simulink library "everscale_lib"  (R2018b)
settings: Solver=VariableStepAuto  StartTime=0.0  StopTime=10.0  RelTol=1e-3
undefined symbols (not defined in the file or in its folder): lindi
libraries: filters_lib x1
settings Model: Creator=Ybeyer  LastModifiedBy=yannic
settings DebuggingCC: LibraryContextMissingDiagnostic=none
settings SFSimCC: SimUseLocalCustomCode=off
settings RTWCC: RTWUseLocalCustomCode=off
settings CodeAppCC: StateflowObjectComments=on

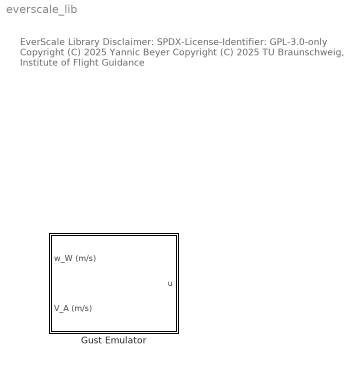
== system everscale_lib ==
  note: EverScale Library
      |
      | Disclaimer:
      | SPDX-License-Identifier: GPL-3.0-only
      |
      | Copyright (C) 2025 Yannic Beyer
      | Copyright (C) 2025 TU Braunschweig, Institute of Flight Guidance
  Gust Emulator : Subsystem  mask{cef=lindi.cef, eig_=lindi.eig}
      mask prompts: cef "Flap control effectiveness struct"; eig_ "Eigendynamics struct"
      mask DialogControl DescGroupVar Prompt: Gust emulator
      mask DialogControl DescTextVar Prompt: This block computes control inputs for an airplane that can emulate the loads of a gust interaction. The gust is specified by a vertical wind speed w_W.

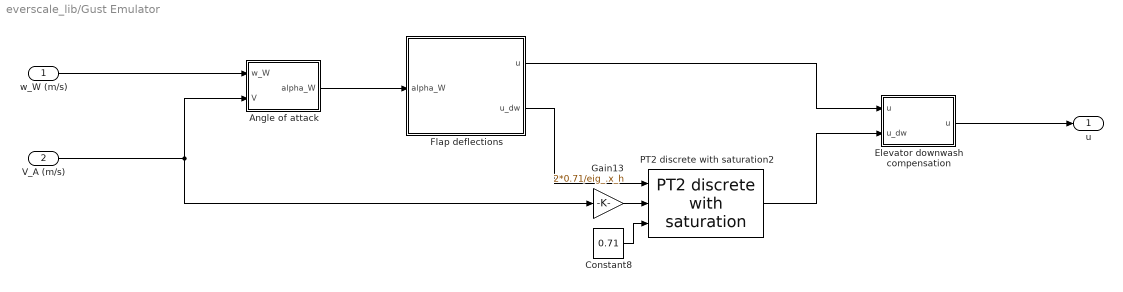
== system everscale_lib/Gust Emulator ==
  w_W (m/s) : Inport
  V_A (m/s) : Inport  Port=2
  Angle of attack : MATLAB Function  TreatAsAtomicUnit=on
  Constant8 : Constant  Value=0.71
  Elevator downwash compensation : MATLAB Function  TreatAsAtomicUnit=on
  Flap deflections : MATLAB Function  TreatAsAtomicUnit=on
  Gain13 : Gain  Gain=2*0.71/eig_.x_h
  PT2 discrete with saturation2 : filters_lib/PT2 discrete with saturation  param_src=external  omega=2/0.035*0.9  d=1  x_max=inf  x_min=-inf  x_dt_max=inf  x_dt_min=-inf  x_dt2_max=inf  x_dt2_min=-inf  y_0_src=internal  x_init=0  y_dt_0_src=internal  x_dt_init=0  is_y_dt_checked=off  is_y_dt2_checked=off  is_external_reset_checked=off  mask_expr_handling_config=default
      settings: SourceProductName=LADAC
  u : Outport
  wires:
  w_W (m/s)/1 -> Angle of attack/1(w_W)
  Flap deflections/2(u_dw) -> PT2 discrete with saturation2/1
  Elevator downwash compensation/1(u) -> u/1
  Angle of attack/1(alpha_W) -> Flap deflections/1(alpha_W)
  Constant8/1 -> PT2 discrete with saturation2/3
  Flap deflections/1(u) -> Elevator downwash compensation/1("u ")
  PT2 discrete with saturation2/1 -> Elevator downwash compensation/2(u_dw)
  V_A (m/s)/1 -> Angle of attack/2(V), Gain13/1
  Gain13/1 -> PT2 discrete with saturation2/2

== matlab function everscale_lib/Gust Emulator/Flap deflections ==
  data: u output; alpha_W input; u_dw output; cef parameter; eig_ parameter
function [u,u_dw] = fcn( alpha_W, cef, eig_)

u = zeros(length(cef.clu),1,class(alpha_W));
clu_w = cef.clu(1:end-2);
dalpha_du = sum(1/eig_.cla*clu_w);
u(1:end-2) = divideFinite(1,dalpha_du)*alpha_W;
u(end-1) = -sum(clu_w.*u(1:end-2)'.*cef.s(1:end-2).*(cef.x(1:end-2)+eig_.xcg-eig_.xnp)) ...
    ./ (cef.clu(end-1)*cef.s(end-1)*(cef.x(end-1)+eig_.xcg-eig_.xnp));

clu_h = cef.clu(end-1);
u_dw_a = divideFinite(1,clu_h)*eig_.cla_h*eig_.dahda*alpha_W;
u_dw_u = -divideFinite(1,clu_h)*eig_.cla_h*eig_.dahdu*u(1:end-2);
u_dw = u_dw_a + u_dw_u;
end

== matlab function everscale_lib/Gust Emulator/Elevator downwash compensation ==
  data: u input; u output; u_dw input
function u = fcn(u,u_dw)
u(end-1) = u(end-1) + u_dw;
end

== matlab function everscale_lib/Gust Emulator/Angle of attack ==
  data: w_W input; alpha_W output; V input
function alpha_W = fcn( w_W, V )
alpha_W = divideFinite( -w_W, V );
end
